simulink subsystem "CONTROLLER_MODEL"  (R2024b)
settings: Solver=VariableStepAuto  StartTime=0.0  StopTime=10.0  RelTol=1e-3
values from neighbouring files (symbols this model uses):
  I = [0.058816667 0 0; 0 0.054000375 0; 0 0 0.011250375]    [Richero280245_Assign2_main.m]
  kd = eps*wn.*diag(I)    [Richero280245_Assign2_main.m]
  kp = diag(I).*wn.^2    [Richero280245_Assign2_main.m]
libraries: vrlib x2, simulink x2
settings Model: Creator=carlorichero  LastModifiedBy=carlorichero

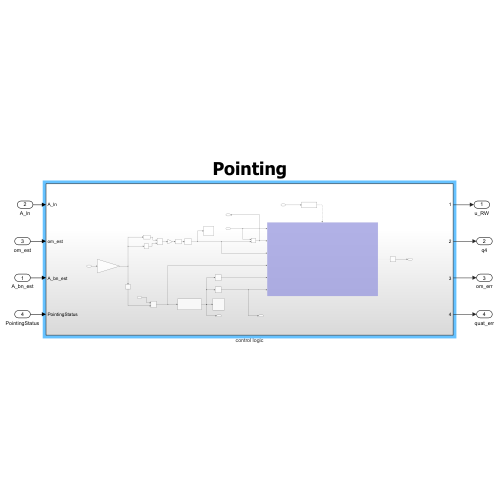
[thumbnail: Simulink's stored preview of the top-level diagram]
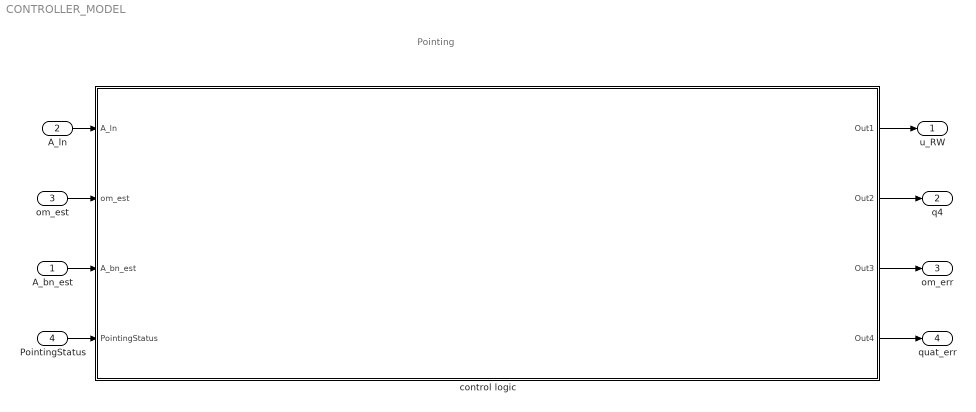
== system CONTROLLER_MODEL ==
  note: Pointing
  A_bn_est : Inport
  A_ln : Inport  Port=2
  om_est : Inport  Port=3
  PointingStatus : Inport  Port=4
  control logic : Subsystem
  u_RW : Outport
  q4 : Outport  Port=2
  om_err : Outport  Port=3
  quat_err : Outport  Port=4
  wires:
  om_est/1 -> control logic/2(om_est)
  control logic/1(Out1) -> u_RW/1
  A_bn_est/1 -> control logic/3(A_bn_est)
  A_ln/1 -> control logic/1(A_ln)
  PointingStatus/1 -> control logic/4(PointingStatus)
  control logic/2(Out2) -> q4/1
  control logic/3(Out3) -> om_err/1
  control logic/4(Out4) -> quat_err/1

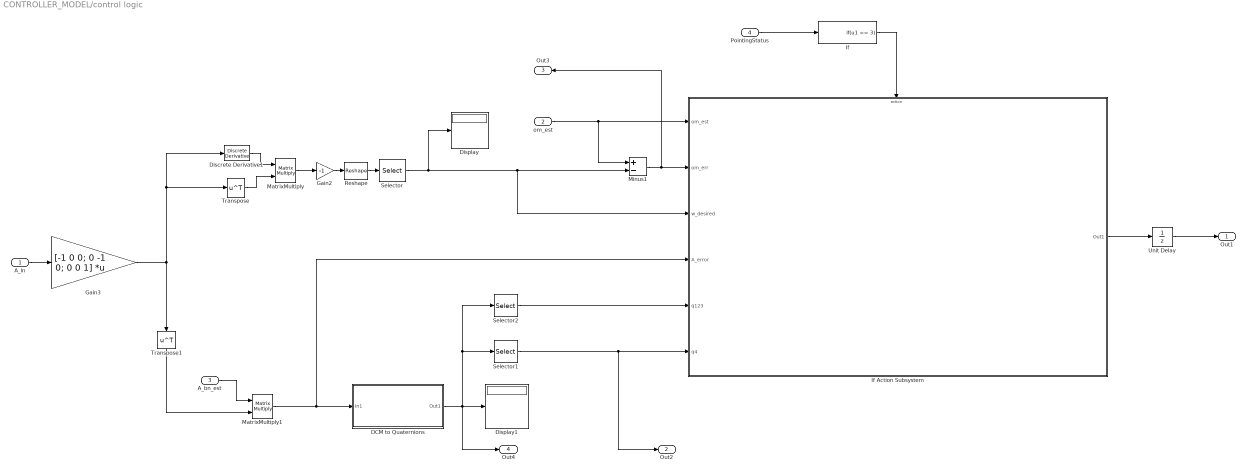
== system CONTROLLER_MODEL/control logic ==
  A_ln : Inport
  om_est : Inport  Port=2
  A_bn_est : Inport  Port=3
  PointingStatus : Inport  Port=4
  DCM to Quaternions : Subsystem
  Discrete Derivative1 : simulink/Discrete/Discrete Derivative  gainval=1.0  ICPrevScaledInput=0.0  OutMin=[]  OutMax=[]  OutDataType=fixdt(1, 16)  OutScaling=2^-10  DoSatur=off
  Display : Display
  Display1 : Display
  Gain2 : Gain  Gain=-1
  Gain3 : Gain  Gain=[-1 0 0; 0 -1 0; 0 0 1]  Multiplication=Matrix(K*u)
  If : If  IfExpression=u1 == 3  ShowElse=off
  If Action Subsystem : Subsystem  TreatAsAtomicUnit=on
  MatrixMultiply : Product  Multiplication=Matrix(*)
  MatrixMultiply1 : Product  Multiplication=Matrix(*)
  Minus1 : Sum  Inputs=+-
  Reshape : Reshape
  Selector : Selector  InputPortWidth=9  IndexOptions=Index vector (dialog)  Indices=[6 7 2]  OutputSizes=1
  Selector1 : Selector  InputPortWidth=4  IndexOptions=Index vector (dialog)  Indices=[4]  OutputSizes=1
  Selector2 : Selector  InputPortWidth=4  IndexOptions=Index vector (dialog)  Indices=[1 2 3]  OutputSizes=1
  Transpose : Math  Operator=transpose
  Transpose1 : Math  Operator=transpose
  Unit Delay : UnitDelay  SampleTime=-1  HasFrameUpgradeWarning=on
  Out1 : Outport
  Out2 : Outport  Port=2
  Out3 : Outport  Port=3
  Out4 : Outport  Port=4
  wires:
  Unit Delay/1 -> Out1/1
  DCM to Quaternions/1(Out1) -> Display1/1, Selector1/1, Selector2/1, Out4/1
  Minus1/1 -> Out3/1, If Action Subsystem/2(om_err)
  Selector1/1 -> If Action Subsystem/6(q4), Out2/1
  If Action Subsystem/1(Out1) -> Unit Delay/1
  If/1 -> If Action Subsystem/Action
  A_bn_est/1 -> MatrixMultiply1/1
  om_est/1 -> If Action Subsystem/1(om_est), Minus1/1
  Discrete Derivative1/1 -> MatrixMultiply/1
  MatrixMultiply1/1 -> DCM to Quaternions/1(In1), If Action Subsystem/4(A_error)
  Gain2/1 -> Reshape/1
  Reshape/1 -> Selector/1
  PointingStatus/1 -> If/1
  Selector/1 -> If Action Subsystem/3(w_desired), Minus1/2, Display/1
  MatrixMultiply/1 -> Gain2/1
  Gain3/1 -> Transpose1/1, Transpose/1, Discrete Derivative1/1
  Selector2/1 -> If Action Subsystem/5(q123)
  Transpose1/1 -> MatrixMultiply1/2
  Transpose/1 -> MatrixMultiply/2
  A_ln/1 -> Gain3/1

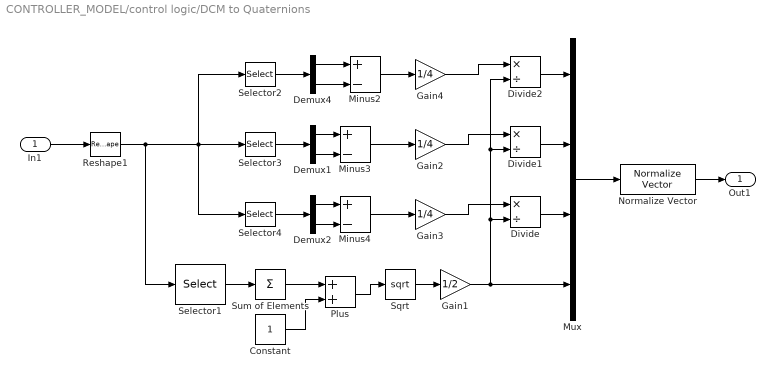
== system CONTROLLER_MODEL/control logic/DCM to Quaternions ==
  In1 : Inport
  Constant : Constant
  Demux1 : Demux  Outputs=2
  Demux2 : Demux  Outputs=2
  Demux4 : Demux  Outputs=2
  Divide : Product  Inputs=*/
  Divide1 : Product  Inputs=*/
  Divide2 : Product  Inputs=*/
  Gain1 : Gain  Gain=1/2
  Gain2 : Gain  Gain=1/4
  Gain3 : Gain  Gain=1/4
  Gain4 : Gain  Gain=1/4
  Minus2 : Sum  Inputs=+-
  Minus3 : Sum  Inputs=+-
  Minus4 : Sum  Inputs=+-
  Mux : Mux
  Normalize Vector : vrlib/Utilities/Normalize Vector  maxzero=0
  Plus : Sum
  Reshape1 : Reshape
  Selector1 : Selector  InputPortWidth=9  IndexOptions=Index vector (dialog)  Indices=[1 5 9]  OutputSizes=1
  Selector2 : Selector  InputPortWidth=9  IndexOptions=Index vector (dialog)  Indices=[8 6]  OutputSizes=1
  Selector3 : Selector  InputPortWidth=9  IndexOptions=Index vector (dialog)  Indices=[3 7]  OutputSizes=1
  Selector4 : Selector  InputPortWidth=9  IndexOptions=Index vector (dialog)  Indices=[4 2]  OutputSizes=1
  Sqrt : Sqrt
  Sum of Elements : Sum  Inputs=+
  Out1 : Outport
  wires:
  Reshape1/1 -> Selector3/1, Selector4/1, Selector2/1, Selector1/1
  Selector1/1 -> Sum of Elements/1
  Normalize Vector/1 -> Out1/1
  Divide2/1 -> Mux/1
  Minus3/1 -> Gain2/1
  Demux2/1 -> Minus4/1
  Demux2/2 -> Minus4/2
  Demux4/1 -> Minus2/1
  Selector3/1 -> Demux1/1
  Mux/1 -> Normalize Vector/1
  Minus2/1 -> Gain4/1
  Sum of Elements/1 -> Plus/1
  In1/1 -> Reshape1/1
  Gain4/1 -> Divide2/1
  Minus4/1 -> Gain3/1
  Divide1/1 -> Mux/2
  Selector2/1 -> Demux4/1
  Demux4/2 -> Minus2/2
  Plus/1 -> Sqrt/1
  Demux1/2 -> Minus3/2
  Divide/1 -> Mux/3
  Constant/1 -> Plus/2
  Demux1/1 -> Minus3/1
  Selector4/1 -> Demux2/1
  Sqrt/1 -> Gain1/1
  Gain1/1 -> Divide/2, Divide1/2, Divide2/2, Mux/4
  Gain2/1 -> Divide1/1
  Gain3/1 -> Divide/1

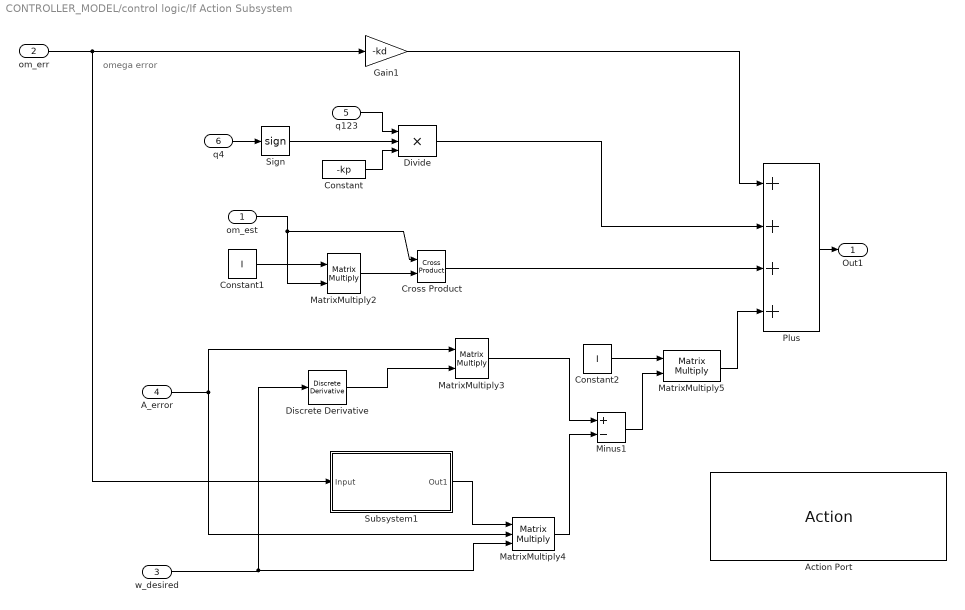
== system CONTROLLER_MODEL/control logic/If Action Subsystem ==
  note: omega
      | error
  om_est : Inport
  om_err : Inport  Port=2
  w_desired : Inport  Port=3
  A_error : Inport  Port=4
  q123 : Inport  Port=5
  q4 : Inport  Port=6
  Action Port : ActionPort
  Constant : Constant  Value=-kp
  Constant1 : Constant  Value=I
  Constant2 : Constant  Value=I
  Cross Product : vrlib/Utilities/Cross Product
  Discrete Derivative : simulink/Discrete/Discrete Derivative  gainval=1.0  ICPrevScaledInput=0.0  OutMin=[]  OutMax=[]  OutDataType=fixdt(1, 16)  OutScaling=2^-10  DoSatur=off
  Divide : Product  Inputs=***
  Gain1 : Gain  Gain=-kd
  MatrixMultiply2 : Product  Multiplication=Matrix(*)
  MatrixMultiply3 : Product  Multiplication=Matrix(*)
  MatrixMultiply4 : Product  Inputs=3  Multiplication=Matrix(*)
  MatrixMultiply5 : Product  Multiplication=Matrix(*)
  Minus1 : Sum  Inputs=+-
  Plus : Sum  Inputs=++++
  Sign : Signum
  Subsystem1 : Subsystem
  Out1 : Outport
  wires:
  q4/1 -> Sign/1
  q123/1 -> Divide/1
  om_err/1 -> Subsystem1/1(Input), Gain1/1
  Constant/1 -> Divide/3
  MatrixMultiply3/1 -> Minus1/1
  A_error/1 -> MatrixMultiply3/1, MatrixMultiply4/2
  Constant2/1 -> MatrixMultiply5/1
  Plus/1 -> Out1/1
  Discrete Derivative/1 -> MatrixMultiply3/2
  Gain1/1 -> Plus/1
  MatrixMultiply5/1 -> Plus/4
  MatrixMultiply2/1 -> Cross Product/2
  Sign/1 -> Divide/2
  Subsystem1/1(Out1) -> MatrixMultiply4/1
  MatrixMultiply4/1 -> Minus1/2
  Constant1/1 -> MatrixMultiply2/1
  Minus1/1 -> MatrixMultiply5/2
  Divide/1 -> Plus/2
  Cross Product/1 -> Plus/3
  om_est/1 -> Cross Product/1, MatrixMultiply2/2
  w_desired/1 -> MatrixMultiply4/3, Discrete Derivative/1

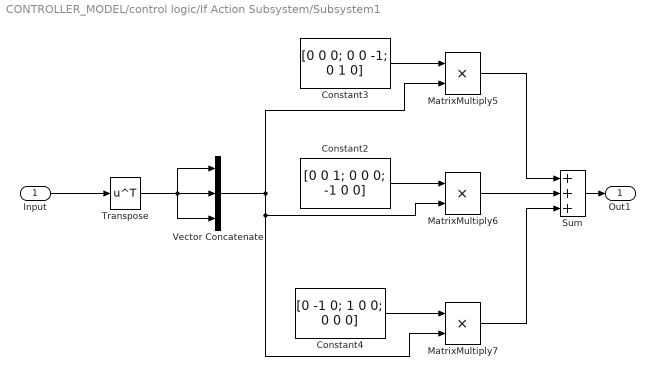
== system CONTROLLER_MODEL/control logic/If Action Subsystem/Subsystem1 ==
  Input : Inport
  Constant2 : Constant  Value=[0 0 1; 0 0 0; -1 0 0]
  Constant3 : Constant  Value=[0 0 0; 0 0 -1; 0 1 0]
  Constant4 : Constant  Value=[0 -1 0; 1 0 0; 0 0 0]
  MatrixMultiply5 : Product
  MatrixMultiply6 : Product
  MatrixMultiply7 : Product
  Sum : Sum  Inputs=+++
  Transpose : Math  Operator=transpose
  Vector Concatenate : Concatenate  NumInputs=3  Mode=Multidimensional array
  Out1 : Outport
  wires:
  Transpose/1 -> Vector Concatenate/1, Vector Concatenate/2, Vector Concatenate/3
  Constant3/1 -> MatrixMultiply5/1
  Vector Concatenate/1 -> MatrixMultiply6/2, MatrixMultiply7/2, MatrixMultiply5/2
  Input/1 -> Transpose/1
  Sum/1 -> Out1/1
  MatrixMultiply6/1 -> Sum/2
  Constant2/1 -> MatrixMultiply6/1
  MatrixMultiply5/1 -> Sum/1
  Constant4/1 -> MatrixMultiply7/1
  MatrixMultiply7/1 -> Sum/3
